simulink model "sim_F450_bare_trim_quaternion"  (R2022a)
settings: Solver=ode4  StartTime=0.0  StopTime=10  FixedStep=0.001  RelTol=1e-3
values from neighbouring files (symbols this model uses):
  u0 = [0.607184471917 2.64116275142e-11 -0.0182106320827 -9.9073551667e-13]    [Qtrim_V5.mat]    (also in Qtrim_hover.mat = [0.608486087464 4.31197561449e-17 4.14393486566e-17 1.124038)
undefined symbols (not defined in the file or in its folder): r2d
settings Model: Creator=ADMIN  LastModifiedBy=USer
settings DebuggingCC: UnconnectedInputMsg=warning  UnconnectedOutputMsg=warning  UnconnectedLineMsg=warning
settings RTWCC: DLArmComputeVersion=19.05

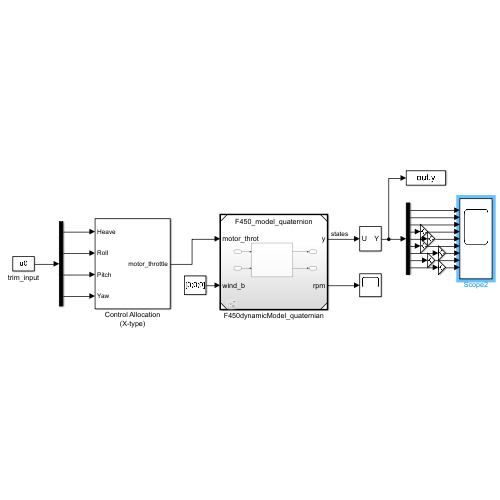
[thumbnail: Simulink's stored preview of the top-level diagram]
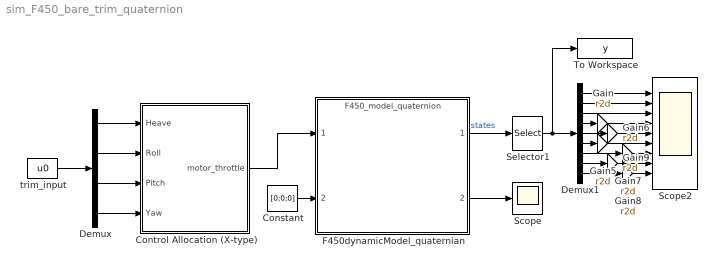
== system sim_F450_bare_trim_quaternion ==
  Constant : Constant  Value=[0;0;0]
  Control Allocation (X-type) : Subsystem
  Demux : Demux
  Demux1 : Demux  Outputs=9
  F450dynamicModel_quaternian : ModelReference  ModelNameDialog=F450_model_quaternion.slx  SimulationMode=Normal  ModelReferenceVersion=10.81
  Gain{,5..9} (6 alike) : Gain  Gain=r2d
  Scope : Scope
  Scope2 : Scope  NumInputPorts=9
  Selector1 : Selector  InputPortWidth=12  IndexOptions=Index vector (dialog)  Indices=1:9  OutputSizes=1
  To Workspace : ToWorkspace  VariableName=y  SampleTime=-1
  trim_input : Constant  Value=u0  OutDataTypeStr=double
  wires:
  Demux/1 -> Control Allocation (X-type)/1(Heave)
  F450dynamicModel_quaternian/2 -> Scope/1
  Control Allocation (X-type)/1(motor_throttle) -> F450dynamicModel_quaternian/1
  Demux1/3 -> Scope2/3
  Demux1/2 -> Scope2/2
  Demux1/4 -> Gain/1
  Demux1/6 -> Gain5/1
  Demux1/9 -> Gain8/1
  Demux1/7 -> Gain7/1
  Demux1/8 -> Gain9/1
  Demux1/5 -> Gain6/1
  Demux1/1 -> Scope2/1
  F450dynamicModel_quaternian/1 -> Selector1/1  "states"
  Gain/1 -> Scope2/4
  Gain6/1 -> Scope2/5
  Gain7/1 -> Scope2/7
  Gain8/1 -> Scope2/9
  Gain9/1 -> Scope2/8
  Gain5/1 -> Scope2/6
  Demux/3 -> Control Allocation (X-type)/3(Pitch)
  Demux/2 -> Control Allocation (X-type)/2(Roll)
  Demux/4 -> Control Allocation (X-type)/4(Yaw)
  trim_input/1 -> Demux/1
  Selector1/1 -> To Workspace/1, Demux1/1
  Constant/1 -> F450dynamicModel_quaternian/2

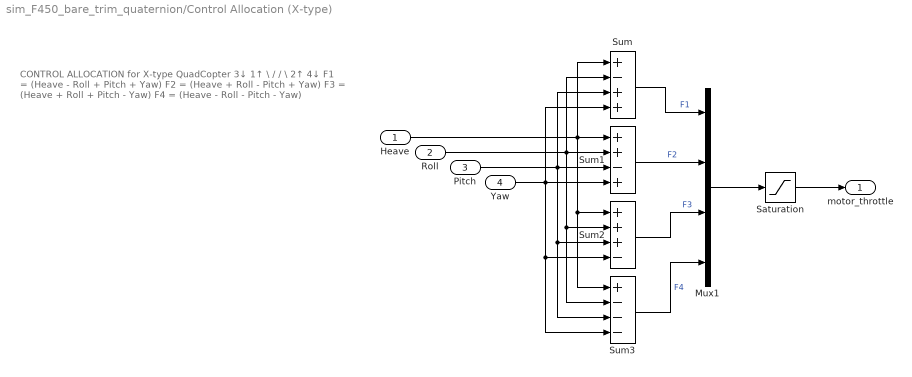
== system sim_F450_bare_trim_quaternion/Control Allocation (X-type) ==
  note: CONTROL ALLOCATION for X-type QuadCopter
      | 3↓ 1↑
      | \ /
      | / \
      | 2↑ 4↓
      | F1 = (Heave - Roll + Pitch + Yaw)
      | F2 = (Heave + Roll - Pitch + Yaw)
      | F3 = (Heave + Roll + Pitch - Yaw)
      | F4 = (Heave - Roll - Pitch - Yaw)
  Heave : Inport
  Roll : Inport  Port=2
  Pitch : Inport  Port=3
  Yaw : Inport  Port=4
  Mux1 : Mux
  Saturation : Saturate  UpperLimit=1  LowerLimit=0
      settings: AttributesFormatString=%<LowerLimit>~%<UpperLimit>
  Sum : Sum  Inputs=+-++
  Sum1 : Sum  Inputs=++-+
  Sum2 : Sum  Inputs=+++-
  Sum3 : Sum  Inputs=+---
  motor_throttle : Outport
  wires:
  Saturation/1 -> motor_throttle/1
  Yaw/1 -> Sum3/4, Sum2/4, Sum/4, Sum1/4
  Pitch/1 -> Sum3/3, Sum2/3, Sum/3, Sum1/3
  Sum3/1 -> Mux1/4  "F4"
  Mux1/1 -> Saturation/1
  Sum1/1 -> Mux1/2  "F2"
  Roll/1 -> Sum3/2, Sum2/2, Sum/2, Sum1/2
  Heave/1 -> Sum3/1, Sum2/1, Sum/1, Sum1/1
  Sum/1 -> Mux1/1  "F1"
  Sum2/1 -> Mux1/3  "F3"
